simulink model "sensor_IMU_model"  (R2025b)
settings: Solver=FixedStepDiscrete  StartTime=0.0  StopTime=10.0  FixedStep=1 / double(IMU_SAMPLE_RATE)  RelTol=1e-3
values from neighbouring files (symbols this model uses):
  IMU_ACC_BIAS : value not decoded    [SensorDict.sldd]
  IMU_ACC_BIAS_WALK = 0.0001    [SensorDict.sldd]
  IMU_ACC_NOISE = 0.001    [SensorDict.sldd]
  IMU_ACC_SCALE = 0.002    [SensorDict.sldd]
  IMU_GYR_BIAS : value not decoded    [SensorDict.sldd]
  IMU_GYR_BIAS_WALK = 1.0E-5    [SensorDict.sldd]
  IMU_GYR_NOISE = 0.0001    [SensorDict.sldd]
  IMU_GYR_SCALE = 0.002    [SensorDict.sldd]
  IMU_SAMPLE_RATE = 1000.0    [SensorDict.sldd]
  IMU_SAT_ACC = 156.96    [SensorDict.sldd]
  IMU_SAT_GYR = 34.907    [SensorDict.sldd]
undefined symbols (not defined in the file or in its folder): DiscIntNeverNeededParam
libraries: simulink x4
settings Model: DataDictionary=SensorDict.sldd  Creator=89447  LastModifiedBy=89447

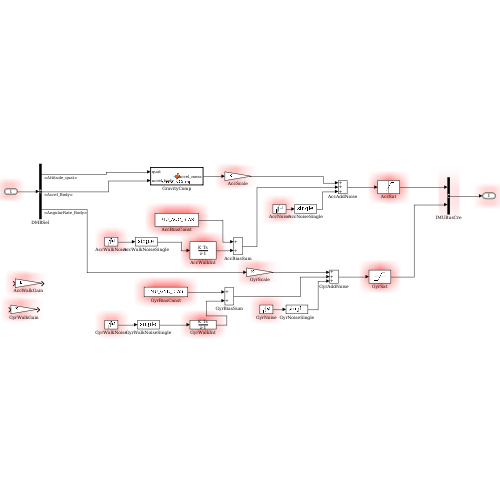
[thumbnail: Simulink's stored preview of the top-level diagram]
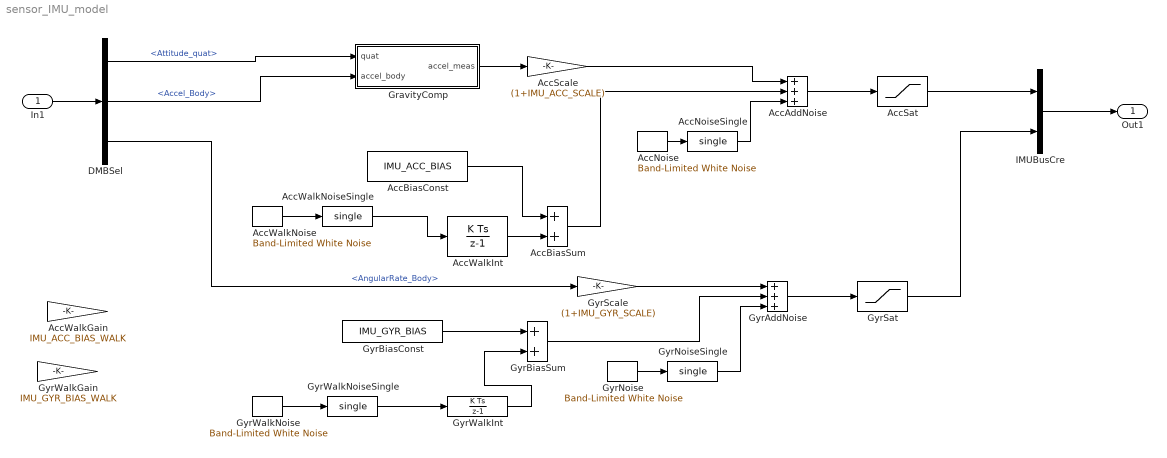
== system sensor_IMU_model ==
  In1 : Inport  OutDataTypeStr=Bus: DynamicModelBus
  AccAddNoise : Sum  Inputs=+++
  AccBiasConst : Constant  Value=IMU_ACC_BIAS
  AccBiasSum : Sum
  AccNoise : simulink/Sources/Band-Limited White Noise  Cov=IMU_ACC_NOISE^2  Ts=1 / double(IMU_SAMPLE_RATE)  seed=[23341]
  AccNoiseSingle : DataTypeConversion  OutDataTypeStr=single  SaturateOnIntegerOverflow=off  RndMeth=Floor
  AccSat : Saturate  UpperLimit=IMU_SAT_ACC  LowerLimit=-IMU_SAT_ACC
  AccScale : Gain  Gain=(1+IMU_ACC_SCALE)
  AccWalkGain : Gain  Gain=IMU_ACC_BIAS_WALK
  AccWalkInt : DiscreteIntegrator  InitialCondition=[0 0 0]  SampleTime=1 / double(IMU_SAMPLE_RATE)  ICPrevOutput=DiscIntNeverNeededParam  ICPrevScaledInput=DiscIntNeverNeededParam
  AccWalkNoise : simulink/Sources/Band-Limited White Noise  Cov=IMU_ACC_BIAS_WALK^2  Ts=1 / double(IMU_SAMPLE_RATE)  seed=[23341]
  AccWalkNoiseSingle : DataTypeConversion  OutDataTypeStr=single  SaturateOnIntegerOverflow=off  RndMeth=Floor
  DMBSel : BusSelector  OutputSignals=Attitude_quat,Accel_Body,AngularRate_Body
  GravityComp : MATLAB Function  TreatAsAtomicUnit=on
  GyrAddNoise : Sum  Inputs=+++
  GyrBiasConst : Constant  Value=IMU_GYR_BIAS
  GyrBiasSum : Sum
  GyrNoise : simulink/Sources/Band-Limited White Noise  Cov=IMU_GYR_NOISE^2  Ts=1 / double(IMU_SAMPLE_RATE)  seed=[23341]
  GyrNoiseSingle : DataTypeConversion  OutDataTypeStr=single  SaturateOnIntegerOverflow=off  RndMeth=Floor
  GyrSat : Saturate  UpperLimit=IMU_SAT_GYR  LowerLimit=-IMU_SAT_GYR
  GyrScale : Gain  Gain=(1+IMU_GYR_SCALE)
  GyrWalkGain : Gain  Gain=IMU_GYR_BIAS_WALK
  GyrWalkInt : DiscreteIntegrator  InitialCondition=[0 0 0]  SampleTime=1 / double(IMU_SAMPLE_RATE)  ICPrevOutput=DiscIntNeverNeededParam  ICPrevScaledInput=DiscIntNeverNeededParam
  GyrWalkNoise : simulink/Sources/Band-Limited White Noise  Cov=IMU_GYR_BIAS_WALK^2  Ts=1 / double(IMU_SAMPLE_RATE)  seed=[23341]
  GyrWalkNoiseSingle : DataTypeConversion  OutDataTypeStr=single  SaturateOnIntegerOverflow=off  RndMeth=Floor
  IMUBusCre : BusCreator  Inputs=2  OutDataTypeStr=Bus: IMU_BUS  NonVirtualBus=on
  Out1 : Outport  OutDataTypeStr=Bus: IMU_BUS
  wires:
  In1/1 -> DMBSel/1
  DMBSel/1 -> GravityComp/1(quat)  "<Attitude_quat>"
  DMBSel/2 -> GravityComp/2(accel_body)  "<Accel_Body>"
  GravityComp/1(accel_meas) -> AccScale/1
  AccScale/1 -> AccAddNoise/1
  AccBiasConst/1 -> AccBiasSum/1
  AccWalkInt/1 -> AccBiasSum/2
  AccBiasSum/1 -> AccAddNoise/2
  AccAddNoise/1 -> AccSat/1
  DMBSel/3 -> GyrScale/1  "<AngularRate_Body>"
  GyrScale/1 -> GyrAddNoise/1
  GyrBiasConst/1 -> GyrBiasSum/1
  GyrWalkInt/1 -> GyrBiasSum/2
  GyrBiasSum/1 -> GyrAddNoise/2
  GyrAddNoise/1 -> GyrSat/1
  AccSat/1 -> IMUBusCre/1
  GyrSat/1 -> IMUBusCre/2
  IMUBusCre/1 -> Out1/1
  AccNoise/1 -> AccNoiseSingle/1
  AccNoiseSingle/1 -> AccAddNoise/3
  AccWalkNoise/1 -> AccWalkNoiseSingle/1
  AccWalkNoiseSingle/1 -> AccWalkInt/1
  GyrNoise/1 -> GyrNoiseSingle/1
  GyrNoiseSingle/1 -> GyrAddNoise/3
  GyrWalkNoise/1 -> GyrWalkNoiseSingle/1
  GyrWalkNoiseSingle/1 -> GyrWalkInt/1

== matlab function sensor_IMU_model/GravityComp ==
  data: quat input; accel_meas output; accel_body input
function accel_meas = GravityComp(quat, accel_body)
%#codegen
% 重力补偿: IMU加速度计测量值 = 体轴加速度 + 重力在体轴投影
% quat: [w,x,y,z] (4x1), accel_body: [ax,ay,az] (3x1)
% accel_meas: IMU实际测量值 (3x1)

g_n = single([0; 0; 9.81]);

% 四元数转旋转矩阵 (手动实现, 代码生成兼容)
q0 = quat(1); q1 = quat(2); q2 = quat(3); q3 = quat(4);
R = single(zeros(3,3));
R(1,1) = 1 - 2*(q2*q2 + q3*q3);
R(1,2) = 2*(q1*q2 - q0*q3);
R(1,3) = 2*(q1*q3 + q0*q2);
R(2,1) = 2*(q1*q2 + q0*q3);
R(2,2) = 1 - 2*(q1*q1 + q3*q3);
R(2,3) = 2*(q2*q3 - q0*q1);
R(3,1) = 2*(q1*q3 - q0*q2);
R(3,2) = 2*(q2*q3 + q0*q1);
R(3,3) = 1 - 2*(q1*q1 + q2*q2);

% 重力在体轴系投影: g_body = R' * g_n
g_body = R' * g_n;

% IMU测量值 = 真实加速度 + 重力分量
accel_meas = accel_body + g_body;
end
